simulink model "example_model"  (R2019b)
settings: Solver=FixedStepDiscrete  StartTime=0.0  StopTime=4000  FixedStep=2  RelTol=1e-3
PreLoadFcn:
  | CreateErrorBuses
  | CreateCyclicFeedbackBuses
  | CreateExtrinsicBuses
  | CreateIntrinsicBuses
  | CreateVisionConfigBuses
  | Simulink.importExternalCTypes('include/kortex_wrapper_data.h');
settings Model: EnablePacing=on  PacingRate=2  Creator=gricher  LastModifiedBy=hlamontagne
settings DataIOCC: ReturnWorkspaceOutputs=off
settings OptimizationCC: EnhancedBackFolding=on  PassReuseOutputArgsAs=Individual arguments  MaxStackSize=64  OptimizeBlockOrder=speed  DifferentSizesBufferReuse=on  OptimizationCustomize=off  EfficientTunableParamExpr=on
settings DebuggingCC: ParameterTunabilityLossMsg=error  ArithmeticOperatorsInVariantConditions=warning
settings HardwareCC: ProdBitPerLong=64  ProdHWDeviceType=Intel->x86-64 (Linux 64)
settings SFSimCC: SimParseCustomCode=off  CustomCodeUndefinedFunction=UseInterfaceOnly
settings RTWCC: SystemTargetFile=ert.tlc  HardwareBoard=Robot Operating System 2 (ROS 2)  TLCOptions=-aInlineSetEventsForThisBaseRateFcn=TLC_FALSE -aSuppressMultiTaskScheduler=TLC_FALSE -aRateBasedStepFcn=1  GenCodeOnly=on  TemplateMakefile=ert_default_tmf  PostCodeGenCommand=kortexPostGeneration(h)  GenerateReport=on  RTWUseSimCustomCode=on  Toolchain=Colcon Tools  IncludeHyperlinkInReport=on  LaunchReport=on  TargetLang=C++  GenerateTraceInfo=on  GenerateTraceReport=on  GenerateTraceReportSl=on  GenerateTraceReportSf=on  GenerateTraceReportEml=on
settings CodeAppCC: ForceParamTrailComments=on  IgnoreCustomStorageClasses=off  OperatorAnnotations=on  SimulinkDataObjDesc=on  SFDataObjDesc=on  InsertBlockDesc=on
settings ERTTargetCC: MultiInstanceERTCode=on  CodeInterfacePackaging=C++ class  SupportVariableSizeSignals=on  RootIOFormat=Structure reference

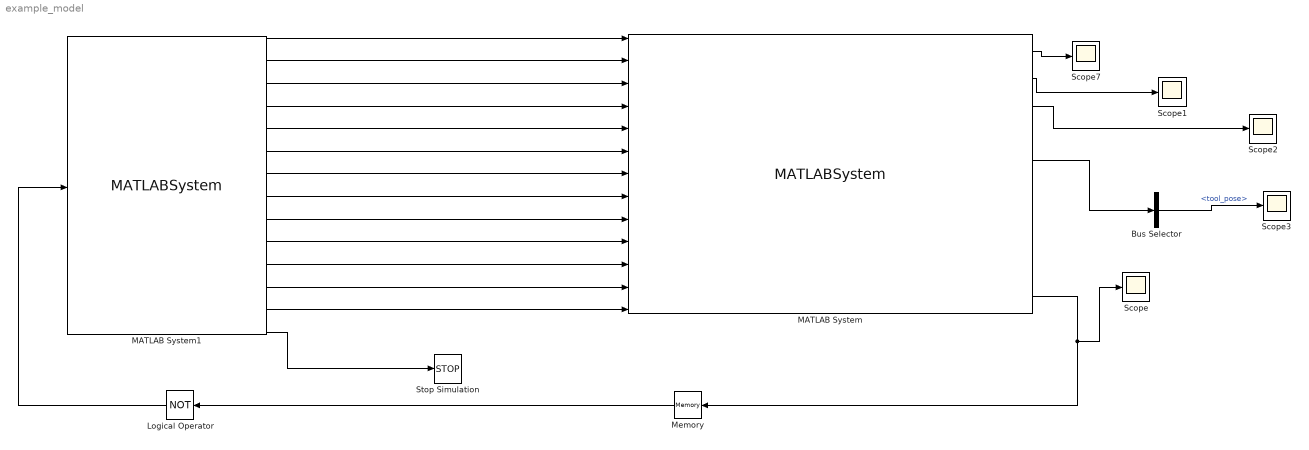
== system example_model ==
  Bus Selector : BusSelector  OutputSignals=tool_pose
  Logical Operator : Logic  Operator=NOT  AllPortsSameDT=off  OutDataTypeStr=boolean
  MATLAB System : MATLABSystem  DialogController=sysobjdialog.BlockDynDialog  System=kortex  nbrJointActuators=6  nbrToolActuators=0  hasVision=true  ip_address=10.0.101.184  user=admin  password=admin  session_connection_timeout=6000000  session_ctrl_timeout=1000000  SimulateUsing=Interpreted execution
      mask Type: kortex
      mask Display:
      | disp('KORTEX Main');
      | port_label('input',1,'cmdToProcess');
      | port_label('input',2,'processCmdSignal');
      | port_label('input',3,'precompute_trj_position');
      | port_label('input',4,'precompute_trj_velocity');
      | port_label('input',5,'precompute_trj_acceleration');
      | port_label('input',6,'precompute_trj_timestamp');
      | port_label('input',7,'precompute_count');
      | port_label('input',8,'joint_constraint');
      | port_label('input',9,'joint_cmd');
      | port_label('input',10,'cartesian_constraint');
      | port_label('input',11,'cartesian_cmd');
      | port_label('input',12,'tool_constraint');
      | port_label('input',13,'tool_cmd');
      | port_label('output',1,'status');
      | port_label('output',2,'cmd_in_progress');
      | port_label('output',3,'moving_status');
      | port_label('output',4,'joint_feedback');
      | port_label('output',5,'base_feedback');
      | port_label('output',6,'tool_feedback');
      | port_label('output',7,'intrinsic_parameters');
      | port_label('output',8,'extrinsic_parameters');
      | port_label('output',9,'vision_settings');
      | port_label('output',10,'is_moving');
  MATLAB System1 : MATLABSystem  System=kObjTrajectoryFeeder  nbrJointActuators=6  SimulateUsing=Interpreted execution
      mask Type: kObjTrajectoryFeeder
      mask Display:
      | disp(['Trajectory' char(10) 'Feeder']);
      | port_label('input',1,'is_ready');
      | port_label('output',1,'cmdToProcess');
      | port_label('output',2,'processCmdSignal');
      | port_label('output',3,'precompute_trj_position');
      | port_label('output',4,'precompute_trj_velocity');
      | port_label('output',5,'precompute_trj_acceleration');
      | port_label('output',6,'precompute_trj_timestamp');
      | port_label('output',7,'precompute_count');
      | port_label('output',8,'joint_constraint');
      | port_label('output',9,'joint_cmd');
      | port_label('output',10,'cartesian_constraint');
      | port_label('output',11,'cartesian_cmd');
      | port_label('output',12,'tool_constraint');
      | port_label('output',13,'tool_cmd');
      | port_label('output',14,'simulation_ended');
  Memory : Memory  InitialCondition=false
  Scope{,1..3,7} (5 alike) : Scope
  Stop Simulation : Stop
  wires:
  Logical Operator/1 -> MATLAB System1/1
  Memory/1 -> Logical Operator/1
  MATLAB System/1 -> Scope7/1
  MATLAB System1/1 -> MATLAB System/1
  MATLAB System1/2 -> MATLAB System/2
  MATLAB System1/3 -> MATLAB System/3
  MATLAB System1/4 -> MATLAB System/4
  MATLAB System1/5 -> MATLAB System/5
  MATLAB System1/6 -> MATLAB System/6
  MATLAB System1/7 -> MATLAB System/7
  MATLAB System1/8 -> MATLAB System/8
  MATLAB System1/14 -> Stop Simulation/1
  MATLAB System/2 -> Scope1/1
  MATLAB System/3 -> Scope2/1
  MATLAB System/10 -> Memory/1, Scope/1
  MATLAB System1/9 -> MATLAB System/9
  MATLAB System1/10 -> MATLAB System/10
  MATLAB System1/11 -> MATLAB System/11
  MATLAB System1/12 -> MATLAB System/12
  MATLAB System1/13 -> MATLAB System/13
  MATLAB System/5 -> Bus Selector/1
  Bus Selector/1 -> Scope3/1  "<tool_pose>"
